simulink model "BPF_Activity3"  (R2022a)
settings: Solver=VariableStepAuto  StartTime=0.0  StopTime=10.0  RelTol=1e-3
values from neighbouring files (symbols this model uses):
  BPF_Sine_Amplitude = 1    [Run_Sim_BPF.m]
  BPF_Sine_Freq = 100    [Run_Sim_BPF.m]
libraries: dsparch4 x4, dspsrcs4 x2
settings Model: Creator=chadw  LastModifiedBy=chadw

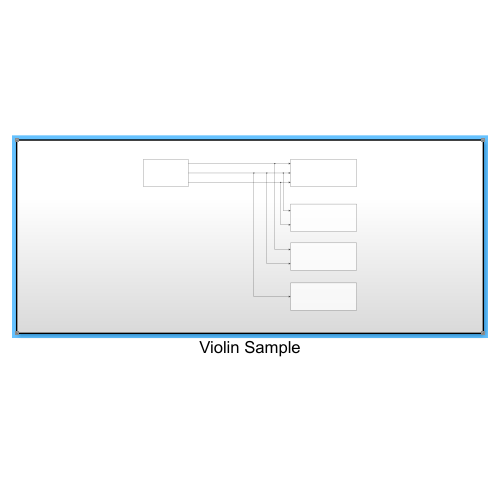
[thumbnail: Simulink's stored preview of the top-level diagram]
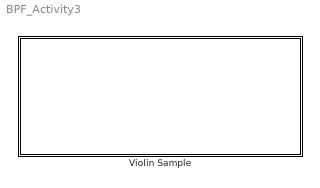
== system BPF_Activity3 ==
  Violin Sample : Subsystem

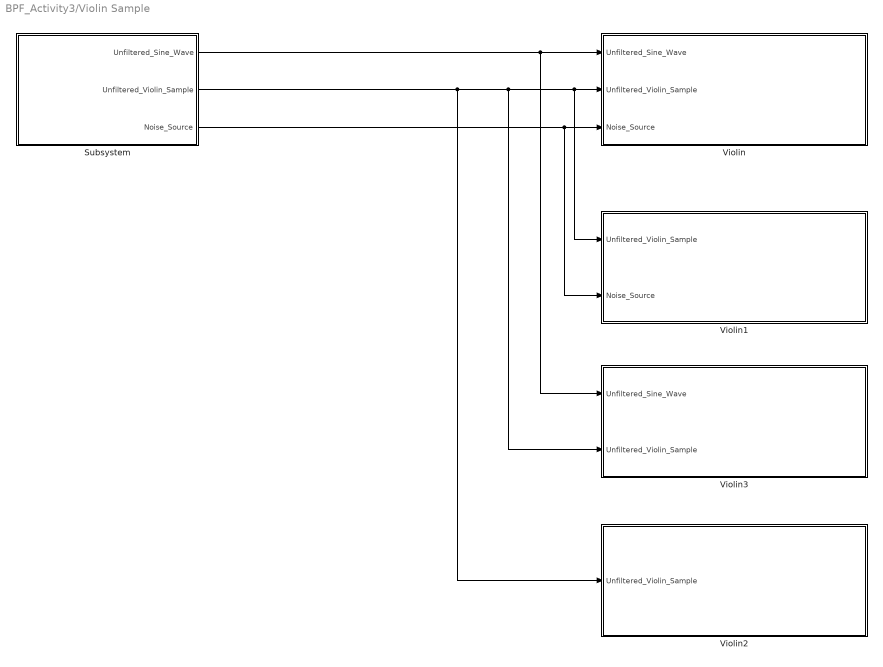
== system BPF_Activity3/Violin Sample ==
  Subsystem : Subsystem
  Violin : Subsystem
  Violin1 : Subsystem
  Violin2 : Subsystem
  Violin3 : Subsystem
  wires:
  Subsystem/2(Unfiltered_Violin_Sample) -> Violin2/1(Unfiltered_Violin_Sample), Violin3/2(Unfiltered_Violin_Sample), Violin1/1(Unfiltered_Violin_Sample), Violin/2(Unfiltered_Violin_Sample)
  Subsystem/1(Unfiltered_Sine_Wave) -> Violin3/1(Unfiltered_Sine_Wave), Violin/1(Unfiltered_Sine_Wave)
  Subsystem/3(Noise_Source) -> Violin1/2(Noise_Source), Violin/3(Noise_Source)

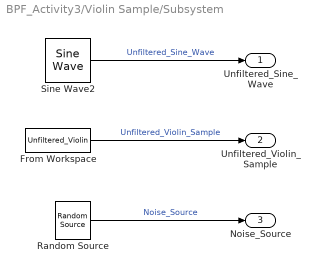
== system BPF_Activity3/Violin Sample/Subsystem ==
  From Workspace : FromWorkspace  VariableName=Unfiltered_Violin  SampleTime=-1
  Random Source : dspsrcs4/Random Source  SrcType=Uniform  NormMethod=Ziggurat  CltLength=12  MinVal=0  MaxVal=1  MeanVal=0  VarVal=1  RepMode=Not repeatable  rawSeed=1  IsInherit=off  SampMode=Discrete  SampTime=1  SampFrame=1  DataType=Double  OutComplex=Real  OutputFrames=off
  Sine Wave2 : dspsrcs4/Sine Wave  Amplitude=BPF_Sine_Amplitude  Frequency=BPF_Sine_Freq  Phase=0  SampleMode=Discrete  OutComplex=Real  CompMethod=Trigonometric fcn  TableSize=Speed  SampleTime=1/1000  SamplesPerFrame=1  ResetState=Restart at time zero  OutputFrames=off  dataType=double  wordLen=16  udDataType=sfix(16)  fracBitsMode=Best precision  numFracBits=15  OutDataTypeStr=double  LastOutDataTypeStr=double
  Unfiltered_Sine_Wave : Outport
  Unfiltered_Violin_Sample : Outport  Port=2
  Noise_Source : Outport  Port=3
  wires:
  Random Source/1 -> Noise_Source/1  "Noise_Source"
  Sine Wave2/1 -> Unfiltered_Sine_Wave/1  "Unfiltered_Sine_Wave"
  From Workspace/1 -> Unfiltered_Violin_Sample/1  "Unfiltered_Violin_Sample"

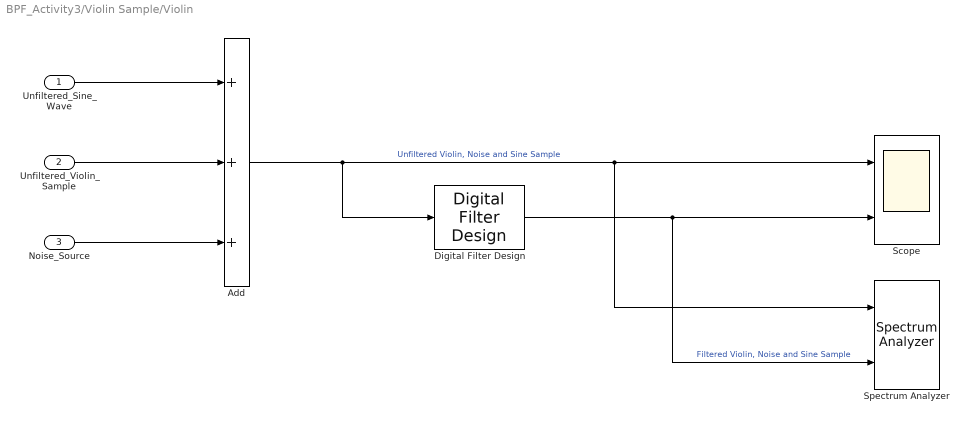
== system BPF_Activity3/Violin Sample/Violin ==
  Unfiltered_Sine_Wave : Inport
  Unfiltered_Violin_Sample : Inport  Port=2
  Noise_Source : Inport  Port=3
  Add : Sum  Inputs=3
  Digital Filter Design : dsparch4/Digital Filter Design  mwdsp_browser_bugfix_var=off
  Scope : Scope  NumInputPorts=2
  Spectrum Analyzer : SpectrumAnalyzer  NumInputPorts=2
  wires:
  Digital Filter Design/1 -> Scope/2, Spectrum Analyzer/2  "Filtered Violin, Noise and Sine Sample"
  Add/1 -> Digital Filter Design/1, Scope/1, Spectrum Analyzer/1  "Unfiltered Violin, Noise and Sine Sample"
  Unfiltered_Sine_Wave/1 -> Add/1
  Unfiltered_Violin_Sample/1 -> Add/2
  Noise_Source/1 -> Add/3

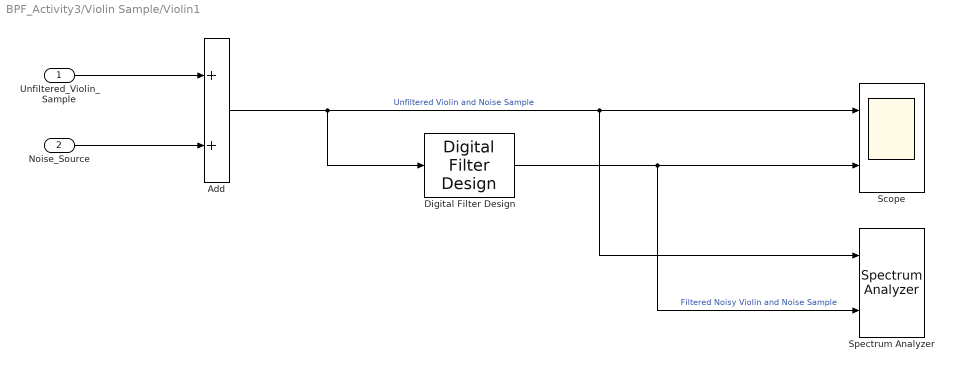
== system BPF_Activity3/Violin Sample/Violin1 ==
  Unfiltered_Violin_Sample : Inport
  Noise_Source : Inport  Port=2
  Add : Sum  Inputs=2
  Digital Filter Design : dsparch4/Digital Filter Design  mwdsp_browser_bugfix_var=off
  Scope : Scope  NumInputPorts=2
  Spectrum Analyzer : SpectrumAnalyzer  NumInputPorts=2
  wires:
  Noise_Source/1 -> Add/2
  Add/1 -> Digital Filter Design/1, Spectrum Analyzer/1, Scope/1  "Unfiltered Violin and Noise Sample"
  Digital Filter Design/1 -> Spectrum Analyzer/2, Scope/2  "Filtered Noisy Violin and Noise Sample"
  Unfiltered_Violin_Sample/1 -> Add/1

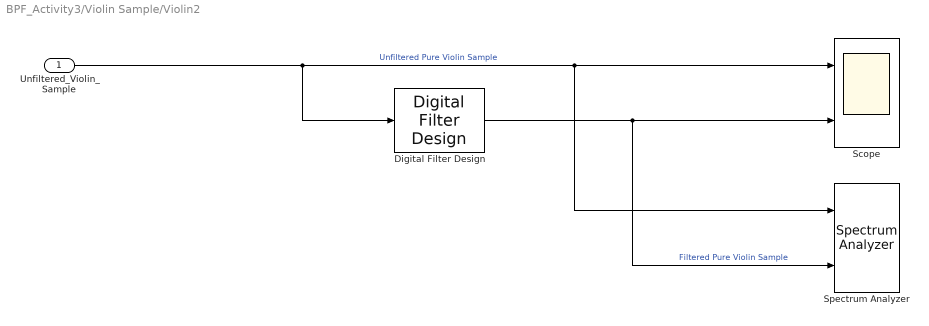
== system BPF_Activity3/Violin Sample/Violin2 ==
  Unfiltered_Violin_Sample : Inport
  Digital Filter Design : dsparch4/Digital Filter Design  mwdsp_browser_bugfix_var=off
  Scope : Scope  NumInputPorts=2
  Spectrum Analyzer : SpectrumAnalyzer  NumInputPorts=2
  wires:
  Digital Filter Design/1 -> Scope/2, Spectrum Analyzer/2  "Filtered Pure Violin Sample"
  Unfiltered_Violin_Sample/1 -> Digital Filter Design/1, Scope/1, Spectrum Analyzer/1  "Unfiltered Pure Violin Sample"

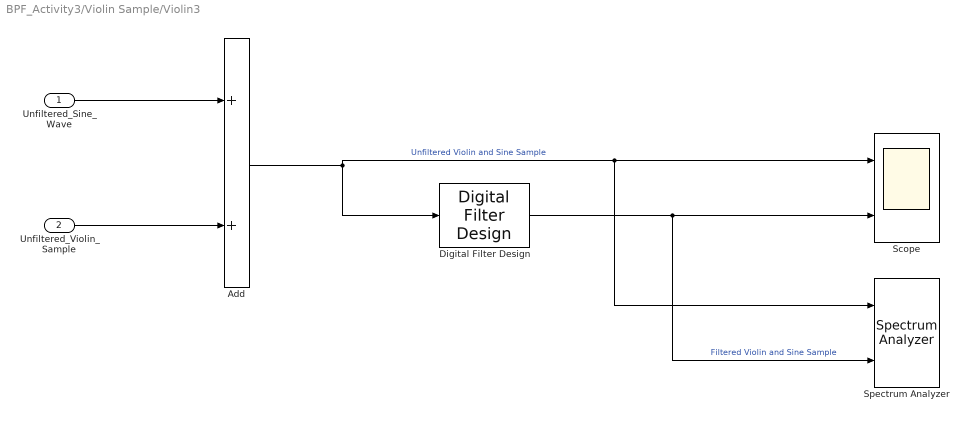
== system BPF_Activity3/Violin Sample/Violin3 ==
  Unfiltered_Sine_Wave : Inport
  Unfiltered_Violin_Sample : Inport  Port=2
  Add : Sum  Inputs=2
  Digital Filter Design : dsparch4/Digital Filter Design  mwdsp_browser_bugfix_var=off
  Scope : Scope  NumInputPorts=2
  Spectrum Analyzer : SpectrumAnalyzer  NumInputPorts=2
  wires:
  Unfiltered_Violin_Sample/1 -> Add/2
  Unfiltered_Sine_Wave/1 -> Add/1
  Add/1 -> Digital Filter Design/1, Spectrum Analyzer/1, Scope/1  "Unfiltered Violin and Sine Sample"
  Digital Filter Design/1 -> Spectrum Analyzer/2, Scope/2  "Filtered Violin and Sine Sample"
